simulink model "freno_motor_carro"  (R2023b)
settings: Solver=VariableStepAuto  StartTime=0.0  StopTime=10.0  RelTol=1e-3
undefined symbols (not defined in the file): btb, Ttb_Max
settings Model: Creator=rodri  LastModifiedBy=rodri

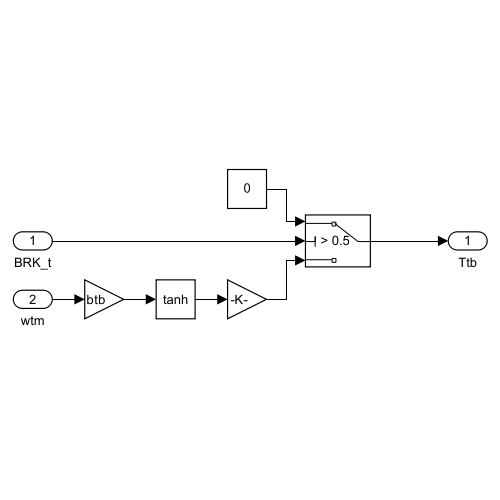
[thumbnail: Simulink's stored preview of the top-level diagram]
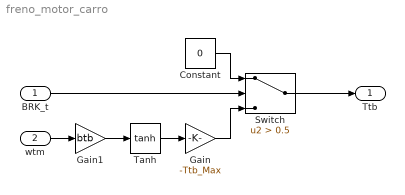
== system freno_motor_carro ==
  BRK_t : Inport
  wtm : Inport  Port=2
  Constant : Constant  Value=0
  Gain : Gain  Gain=-Ttb_Max
  Gain1 : Gain  Gain=btb
  Switch : Switch  Criteria=u2 > Threshold  Threshold=0.5  SaturateOnIntegerOverflow=off  InputSameDT=off
  Tanh : Trigonometry  Operator=tanh
  Ttb : Outport
  wires:
  BRK_t/1 -> Switch/2
  wtm/1 -> Gain1/1
  Switch/1 -> Ttb/1
  Gain1/1 -> Tanh/1
  Tanh/1 -> Gain/1
  Constant/1 -> Switch/1
  Gain/1 -> Switch/3
